simulink model "integracion_motor"  (R2024a)
settings: Solver=VariableStepAuto  StartTime=0.0  StopTime=10  RelTol=1e-3
model workspace (MAT data in the model file):
  kpti = Simulink.Parameter
  kpti.Complexity = 'real'
  kpti.Dimensions = [0 0]
  kpti.DataType = 'auto'
undefined symbols (not defined in the file): kp, LF, t_s, ti
libraries: instrumentseriallib x3
settings Model: Creator=basti  LastModifiedBy=basti

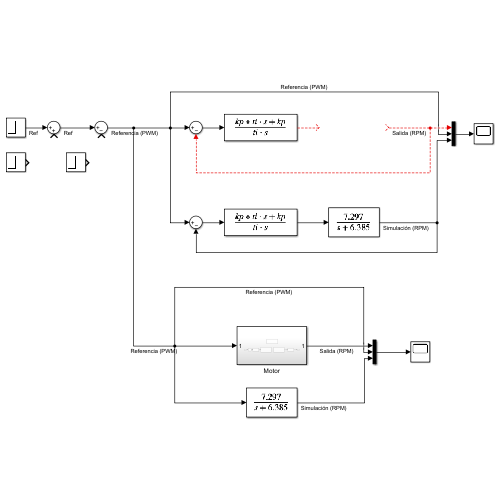
[thumbnail: Simulink's stored preview of the top-level diagram]
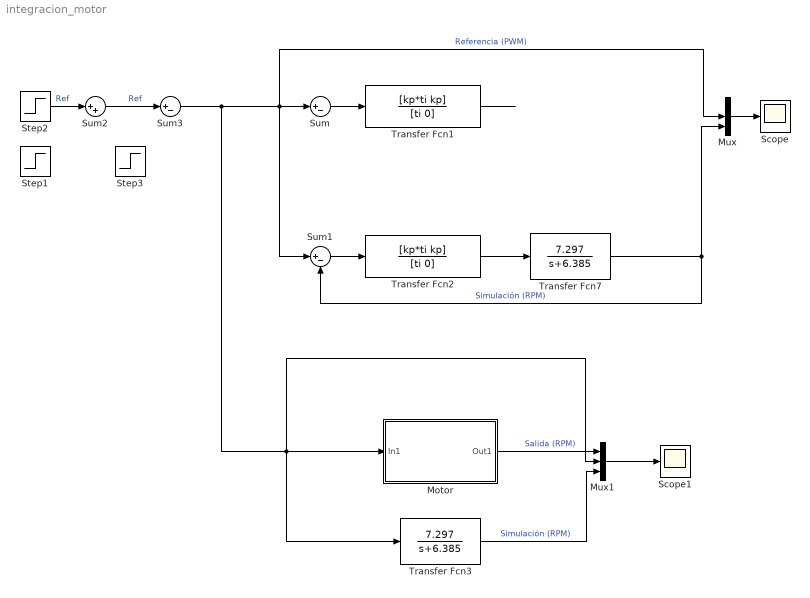
== system integracion_motor ==
  Motor : Subsystem
  Mux : Mux  Inputs=3
  Mux1 : Mux  Inputs=3
  Scope : Scope
  Scope1 : Scope
  Step1 : Step  Time=4  After=10  SampleTime=0
  Step2 : Step  Time=2  After=50  SampleTime=0
  Step3 : Step  Time=6  After=80  SampleTime=0
  Sum : Sum  Inputs=|+-
  Sum1 : Sum  Inputs=|+-
  Sum2 : Sum  Inputs=|++
  Sum3 : Sum  Inputs=|+-
  Transfer Fcn1 : TransferFcn  Numerator=[kp*ti kp]  Denominator=[ti 0]
  Transfer Fcn2 : TransferFcn  Numerator=[kp*ti kp]  Denominator=[ti 0]
  Transfer Fcn3 : TransferFcn  Numerator=[7.297]  Denominator=[1 6.385]
  Transfer Fcn7 : TransferFcn  Numerator=[7.297]  Denominator=[1 6.385]
  wires:
  ? -> Mux/1, Sum/2  "Salida (RPM)"
  Mux/1 -> Scope/1
  Transfer Fcn7/1 -> Sum1/2, Mux/3  "Simulación (RPM)"
  Sum/1 -> Transfer Fcn1/1
  Sum1/1 -> Transfer Fcn2/1
  Transfer Fcn1/1 -> ?
  Transfer Fcn2/1 -> Transfer Fcn7/1
  Sum3/1 -> Motor/1(In1), Transfer Fcn3/1, Mux1/2, Sum1/1, Mux/2, Sum/1  "Referencia (PWM)"
  Motor/1(Out1) -> Mux1/1  "Salida (RPM)"
  Mux1/1 -> Scope1/1
  Transfer Fcn3/1 -> Mux1/3  "Simulación (RPM)"
  Sum2/1 -> Sum3/1  "Ref"
  Step2/1 -> Sum2/1  "Ref"

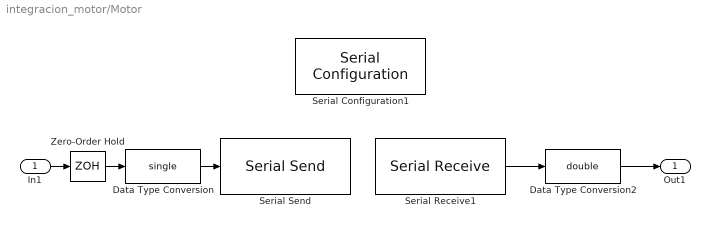
== system integracion_motor/Motor ==
  In1 : Inport
  Data Type Conversion : DataTypeConversion  OutDataTypeStr=single  SaturateOnIntegerOverflow=off  RndMeth=Floor
  Data Type Conversion2 : DataTypeConversion  OutDataTypeStr=double  RndMeth=Nearest  SaturateOnIntegerOverflow=off
  Serial Configuration1 : instrumentseriallib/Serial Configuration  Priority=-200000  PortSel=COM3  Port=COM3  ComPort=COM3  BaudRate=115200  DataBits=8  Parity=none  StopBits=1  ByteOrder=little-endian  FlowControl=none  Timeout=10  SimulateUsing=Interpreted execution  BlockInModel=on  aMode=1
  Serial Receive1 : instrumentseriallib/Serial Receive  Priority=1  PortSel=COM3  Port=COM3  ComPort=COM3  DataType=single  SaveDataType=uint8  ToggleHeader=on  Header='V'  ToggleDataSize=on  DataSize=[1 1]  ToggleTerminator=on  Terminator=LF ('\n')  CustomTerminator=[]  InputFormat=Column major  EnableBlockingMode=on  ActionDataUnavailable=Output last received value  ActionWhenDataUnavailable=Output last received value  CustomValue=0  SampleTime=t_s  SimulateUsing=Interpreted execution  BlockInModel=on  aMode=1
  Serial Send : instrumentseriallib/Serial Send  Priority=1  PortSel=COM3  Port=COM3  ComPort=COM3  Header=[]  Terminator=LF ('\n')  CustomTerminator=[]  EnableBlockingMode=on  SimulateUsing=Interpreted execution  BlockInModel=on  aMode=1
  Zero-Order Hold : ZeroOrderHold  SampleTime=t_s
  Out1 : Outport
  wires:
  In1/1 -> Zero-Order Hold/1
  Zero-Order Hold/1 -> Data Type Conversion/1
  Data Type Conversion/1 -> Serial Send/1
  Serial Receive1/1 -> Data Type Conversion2/1
  Data Type Conversion2/1 -> Out1/1
